simulink model "ec_fixed_slm_hardcode"  (Simulink 10.0)
settings: Solver=FixedStepDiscrete  StartTime=0.0  StopTime=10  RelTol=1e-3
libraries: dspsrcs4 x14, simulink x8, dspsnks4 x4, dspsigops x2, dspbuff3 x2, dspadpt3 x1
settings Model: Creator=Kerry Schutz  LastModifiedBy=bhisma
settings DataIOCC: LimitDataPoints=on  SignalLoggingSaveFormat=ModelDataLogs
settings OptimizationCC: BlockReduction=off  DefaultParameterBehavior=Inlined  InlineInvariantSignals=on  ExpressionDepthLimit=2147483647  StateBitsets=on  DataBitsets=on  ZeroExternalMemoryAtStartup=off  ZeroInternalMemoryAtStartup=off  EfficientFloat2IntCast=on  LifeSpan=1  EfficientTunableParamExpr=on
settings DebuggingCC: AlgebraicLoopMsg=none  SaveWithParameterizedLinksMsg=none  SolverPrmCheckMsg=warning  FcnCallInpInsideContextMsg=warning  StateNameClashWarn=warning
settings HardwareCC: ProdBitPerInt=16  ProdBitPerPointer=16  ProdBitPerSizeT=16  ProdBitPerPtrDiffT=16  ProdIntDivRoundTo=Zero  ProdEndianess=LittleEndian  ProdWordSize=16  ProdHWDeviceType=Microchip->dsPIC  TargetBitPerInt=16  TargetIntDivRoundTo=Zero  TargetEndianess=LittleEndian  TargetWordSize=16  TargetHWDeviceType=Microchip->dsPIC
settings SFSimCC: SimUseLocalCustomCode=on  SimParseCustomCode=off  MATLABDynamicMemAlloc=off  CustomCodeUndefinedFunction=FilterOut
settings RTWCC: Description=Real-Time Workshop Embedded Coder (no auto configuration)  SystemTargetFile=ert.tlc  GenCodeOnly=on  TemplateMakefile=ert_default_tmf  RTWUseLocalCustomCode=on  PortableWordSizes=on  CreateSILPILBlock=SIL
settings CodeAppCC: IgnoreCustomStorageClasses=off  CustomSymbolStrType=$N$R$M  InternalIdentifier=Classic  InlinedPrmAccess=Macros
settings ERTTargetCC: TargetFcnLib=ansi_tfl_tmw.mat  GenerateSampleERTMain=on  IncludeMdlTerminateFcn=off  SupportAbsoluteTime=off  PurelyIntegerCode=on  SupportNonFinite=off  SupportComplex=off  InlinedParameterPlacement=NonHierarchical  ERTCustomFileTemplate=example_file_process.tlc  ConvertIfToSwitch=off  SuppressUnreachableDefaultCases=off

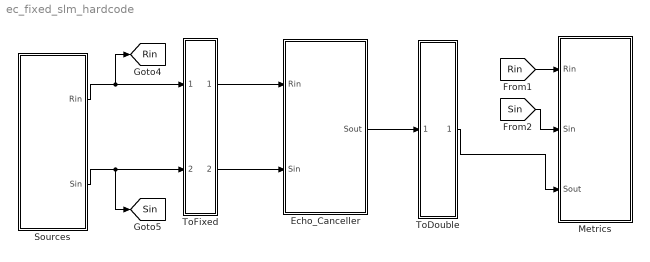
== system ec_fixed_slm_hardcode ==
  Echo_Canceller : Subsystem
  Metrics : Subsystem  TreatAsAtomicUnit=on
  Sources : Subsystem
  ToDouble : Subsystem
  ToFixed : Subsystem
  tag scope: Rin=global, Sin=global
  wires:
  ToFixed/1(Rin) -> Echo_Canceller/1(Rin)
  ToFixed/2(Sin) -> Echo_Canceller/2("Sin ")
  Echo_Canceller/1(Sout) -> ToDouble/1(In2)
  Sources/2(Sin) -> ToFixed/2(" In2"), [Sin]
  Sources/1(Rin) -> ToFixed/1(In1), [Rin]
  [Rin] -> Metrics/1(Rin)
  [Sin] -> Metrics/2(Sin)
  ToDouble/1(Sout) -> Metrics/3(Sout)

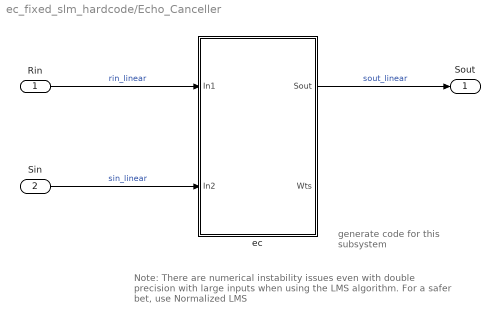
== system ec_fixed_slm_hardcode/Echo_Canceller ==
  note: Note:
      | There are numerical instability issues even with double precision
      | with large inputs when using the LMS algorithm.
      | For a safer bet, use Normalized LMS
  note: generate code for this
      | subsystem
  Rin : Inport
  "Sin " : Inport  Port=2
  ec : Subsystem
  Sout : Outport
  wires:
  Rin/1 -> ec/1(In1)  "rin_linear"
  "Sin "/1 -> ec/2(In2)  "sin_linear"
  ec/1(Sout) -> Sout/1  "sout_linear"

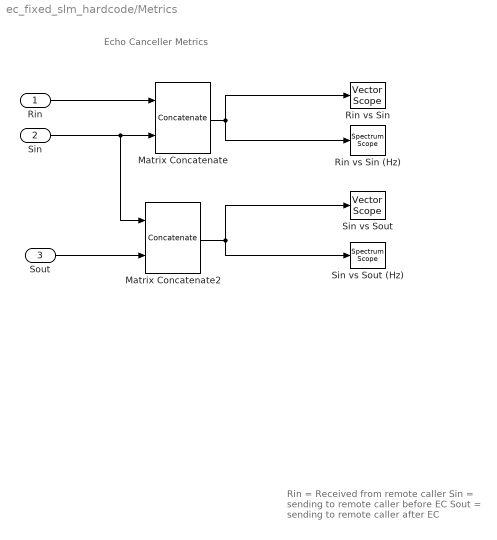
== system ec_fixed_slm_hardcode/Metrics ==
  note: Rin = Received from remote caller
      | Sin = sending to remote caller before EC
      | Sout = sending to remote caller after EC
  note: Echo Canceller Metrics
  Rin : Inport
  Sin : Inport  Port=2
  Sout : Inport  Port=3
  Matrix Concatenate : Concatenate  Mode=Multidimensional array  ConcatenateDimension=2
  Matrix Concatenate2 : Concatenate  Mode=Multidimensional array  ConcatenateDimension=2
  Rin vs Sin : dspsnks4/Vector Scope  ScopeProperties=on  Domain=Time  HorizSpan=1  DisplayProperties=off  AxisGrid=on  Memory=off  FrameNumber=on  AxisLegend=off  AxisZoom=off  OpenScopeAtSimStart=on  OpenScopeImmediately=off  FigPos=[21 752 407 182]  AxisProperties=off  XUnits=Hertz  XRange=[0...Fs/2]  InheritXIncr=on  XIncr=1  XLabel=Time  XLimit=Auto  XMin=0  XMax=1  XStart=0  YUnits=dB  YLabel=Amplitude  LineProperties=off  LineColors=[1 0 0]|[0 1 0]
      settings: SourceProductName=DSP System Toolbox  SourceProductBaseCode=DS  YMin=-1  YMax=1
  Rin vs Sin (Hz) : dspsnks4/Spectrum Scope  SystemSampleTime=-1  ScopeProperties=on  Domain=Frequency  HorizSpan=1  UseBuffer=on  BufferSize=512  Overlap=64  inpFftLenInherit=off  FFTlength=128  numAvg=2  DisplayProperties=off  AxisGrid=on  Memory=off  FrameNumber=on  AxisLegend=off  AxisZoom=off  OpenScopeAtSimStart=on  OpenScopeImmediately=off  FigPos=[22 519 408 178]  AxisProperties=off  XUnits=Hertz  XRange=[0...Fs/2]  InheritXIncr=on  XIncr=1.0  XLabel=Samples  XLimit=Auto  YUnits=dB  XMax=1  XMin=0  YLabel=Magnitude-squared, dB  LineProperties=off  LineColors=[1 0 0]|[0 1 0]  wintypeSpecScope=Hann  RsSpecScope=50  betaSpecScope=5  winsampSpecScope=Periodic
      settings: SourceProductName=DSP System Toolbox  SourceProductBaseCode=DS  YMin=-87.2863320440191  YMax=22.6100164436924
  Sin vs Sout : dspsnks4/Vector Scope  ScopeProperties=on  Domain=Time  HorizSpan=1  DisplayProperties=off  AxisGrid=on  Memory=off  FrameNumber=on  AxisLegend=off  AxisZoom=off  OpenScopeAtSimStart=on  OpenScopeImmediately=off  FigPos=[439 284 406 181]  AxisProperties=off  XUnits=Hertz  XRange=[0...Fs/2]  InheritXIncr=on  XIncr=1  XLabel=Time  XLimit=Auto  XMin=0  XMax=1  XStart=0  YUnits=dB  YLabel=Amplitude  LineProperties=off  LineColors=[1 0 0]|[0 1 0]
      settings: SourceProductName=DSP System Toolbox  SourceProductBaseCode=DS  YMin=-1.10854137455551  YMax=1.10983865900285
  Sin vs Sout (Hz) : dspsnks4/Spectrum Scope  SystemSampleTime=-1  ScopeProperties=on  Domain=Frequency  HorizSpan=1  UseBuffer=on  BufferSize=512  Overlap=64  inpFftLenInherit=off  FFTlength=128  numAvg=2  DisplayProperties=off  AxisGrid=on  Memory=off  FrameNumber=on  AxisLegend=off  AxisZoom=off  OpenScopeAtSimStart=on  OpenScopeImmediately=off  FigPos=[440 519 404 181]  AxisProperties=off  XUnits=Hertz  XRange=[0...Fs/2]  InheritXIncr=on  XIncr=1.0  XLabel=Samples  XLimit=Auto  YUnits=dB  XMax=1  XMin=0  YLabel=Magnitude-squared, dB  LineProperties=off  LineColors=[1 0 0]|[0 1 0]  wintypeSpecScope=Hann  RsSpecScope=50  betaSpecScope=5  winsampSpecScope=Periodic
      settings: SourceProductName=DSP System Toolbox  SourceProductBaseCode=DS  YMin=-128.562839071617  YMax=21.0948472865104
  wires:
  Sout/1 -> Matrix Concatenate2/2
  Matrix Concatenate2/1 -> Sin vs Sout/1, Sin vs Sout (Hz)/1
  Matrix Concatenate/1 -> Rin vs Sin/1, Rin vs Sin (Hz)/1
  Rin/1 -> Matrix Concatenate/1
  Sin/1 -> Matrix Concatenate/2, Matrix Concatenate2/1

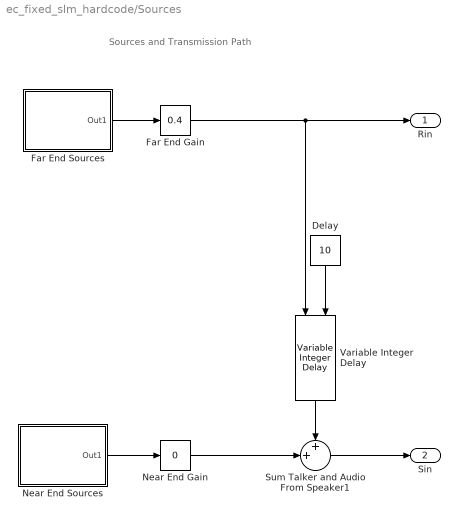
== system ec_fixed_slm_hardcode/Sources ==
  note: Sources and Transmission Path
  Delay : Constant  Value=10  SampleTime=80/8000
  Far End Gain : simulink/Math Operations/Slider Gain  SystemSampleTime=-1  low=0  gain=0.4  high=10
  Far End Sources : Subsystem
  Near End Gain : simulink/Math Operations/Slider Gain  SystemSampleTime=-1  low=0  gain=0  high=10
  Near End Sources : Subsystem
  Sum Talker and Audio From Speaker1 : Sum  Inputs=++|  SaturateOnIntegerOverflow=on  InputSameDT=on  OutDataTypeStr=Inherit: Same as first input
  Variable Integer Delay : dspsigops/Variable Integer Delay  dmax=100  ic=0
      settings: SourceProductName=DSP System Toolbox  SourceProductBaseCode=DS
  Rin : Outport
  Sin : Outport  Port=2
  wires:
  Far End Gain/1 -> Rin/1, Variable Integer Delay/1
  Near End Gain/1 -> Sum Talker and Audio From Speaker1/2
  Near End Sources/1(Out1) -> Near End Gain/1
  Far End Sources/1(Out1) -> Far End Gain/1
  Sum Talker and Audio From Speaker1/1 -> Sin/1
  Variable Integer Delay/1 -> Sum Talker and Audio From Speaker1/1
  Delay/1 -> Variable Integer Delay/2

== system ec_fixed_slm_hardcode/ToDouble ==
  In2 : Inport
  " 6" : DataTypeConversion  OutDataTypeStr=double
  Sout : Outport
  wires:
  In2/1 -> " 6"/1
  " 6"/1 -> Sout/1

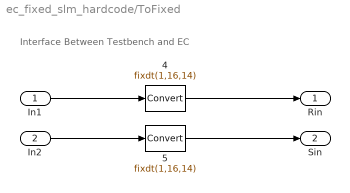
== system ec_fixed_slm_hardcode/ToFixed ==
  note: Interface Between Testbench and EC
  In1 : Inport
  " In2" : Inport  Port=2
  " 4" : DataTypeConversion  OutDataTypeStr=fixdt(1,16,14)
  " 5" : DataTypeConversion  OutDataTypeStr=fixdt(1,16,14)
  Rin : Outport
  Sin : Outport  Port=2
  wires:
  In1/1 -> " 4"/1
  " In2"/1 -> " 5"/1
  " 4"/1 -> Rin/1
  " 5"/1 -> Sin/1

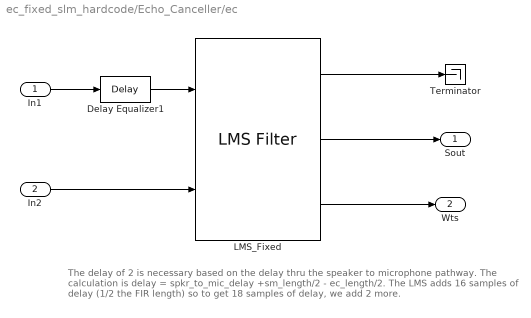
== system ec_fixed_slm_hardcode/Echo_Canceller/ec ==
  note: The delay of 2 is necessary based on the delay thru the speaker to microphone pathway.
      | The calculation is delay = spkr_to_mic_delay +sm_length/2 - ec_length/2. The LMS
      | adds 16 samples of delay (1/2 the FIR length) so to get 18 samples of delay, we add 2 more.
  In1 : Inport
  In2 : Inport  Port=2
  Delay Equalizer1 : dspsigops/Delay  dly_unit=Samples  delay=2  ic_detail=off  dif_ic_for_ch=off  dif_ic_for_dly=off  ic=0  reset_popup=None
      settings: SourceProductName=DSP System Toolbox  SourceProductBaseCode=DS
  LMS_Fixed : dspadpt3/LMS Filter  Algo=LMS  L=32  stepflag=Dialog  mu=300/32768  leakage=1  ic=0  Adapt=off  resetflag=None  weights=on  secondCoeffMode=User-defined  secondCoeffWordLength=2  secondCoeffFracLength=14  accumMode=Binary point scaling  accumWordLength=16  accumFracLength=20  accum2Mode=User-defined  accum2FracLength=15  prodOutputMode=Binary point scaling  prodOutputWordLength=16  prodOutputFracLength=20  prodOutput2Mode=User-defined  prodOutput2FracLength=15  prodOutput3Mode=User-defined  prodOutput3FracLength=15  prodOutput4Mode=User-defined  prodOutput4FracLength=15  quotientMode=User-defined  quotientFracLength=20  memoryMode=Binary point scaling  memoryWordLength=16  memoryFracLength=15  roundingMode=Nearest  overflowMode=off  addnparflag=off
      settings: SourceProductName=DSP System Toolbox  SourceProductBaseCode=DS
  Terminator : Terminator
  Sout : Outport
  Wts : Outport  Port=2
  wires:
  Delay Equalizer1/1 -> LMS_Fixed/1
  LMS_Fixed/3 -> Wts/1
  LMS_Fixed/2 -> Sout/1
  In2/1 -> LMS_Fixed/2
  LMS_Fixed/1 -> Terminator/1
  In1/1 -> Delay Equalizer1/1

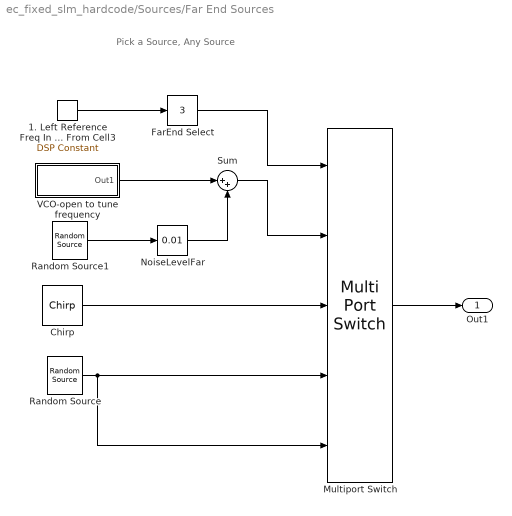
== system ec_fixed_slm_hardcode/Sources/Far End Sources ==
  note: Pick a Source, Any Source
  1. Left Reference Freq In Hz From Cell3 : dspsrcs4/DSP Constant  SystemSampleTime=-1  Value=1  SampleMode=Discrete  discreteOutput=Sample-based  continuousOutput=Sample-based  sampTime=1/8000  framePeriod=2  dataType=double  isSigned=on  wordLen=16  udDataType=sfix(16)  fracBitsMode=Best precision  numFracBits=15  InterpretAs1D=-inf  Ts=-inf  FramebasedOutput=-inf
      settings: SourceProductName=DSP System Toolbox  SourceProductBaseCode=DS  additionalParams=on
  Chirp : dspsrcs4/Chirp  sweep=Linear  mode=Unidirectional  f0=100  f1=4000  t1=80/8000  Tsweep=80/8000  phase=0  Ts=1/8000  spf=80  datatype=Double
      settings: SourceProductName=DSP System Toolbox
  FarEnd Select : simulink/Math Operations/Slider Gain  SystemSampleTime=-1  low=0  gain=3  high=10
  Multiport Switch : MultiPortSwitch  Inputs=4  SampleTime=80/8000
  NoiseLevelFar : simulink/Math Operations/Slider Gain  SystemSampleTime=-1  low=0  gain=0.01  high=1
  Random Source : dspsrcs4/Random Source  SrcType=Gaussian  NormMethod=Ziggurat  CltLength=12  MinVal=0  MaxVal=1  MeanVal=0  VarVal=1  RepMode=Repeatable  rawSeed=1  IsInherit=off  SampMode=Discrete  SampTime=1/8000  SampFrame=80  DataType=Double  OutComplex=Real
  Random Source1 : dspsrcs4/Random Source  SrcType=Gaussian  NormMethod=Ziggurat  CltLength=12  MinVal=0  MaxVal=1  MeanVal=0  VarVal=1  RepMode=Not repeatable  rawSeed=1  IsInherit=off  SampMode=Discrete  SampTime=1/8000  SampFrame=80  DataType=Double  OutComplex=Real
  Sum : Sum  Inputs=|++
  VCO-open to tune frequency : Subsystem
  Out1 : Outport
  wires:
  VCO-open to tune frequency/1(Out1) -> Sum/1
  Multiport Switch/1 -> Out1/1
  Chirp/1 -> Multiport Switch/3
  Random Source/1 -> Multiport Switch/4, Multiport Switch/5
  1. Left Reference Freq In Hz From Cell3/1 -> FarEnd Select/1
  FarEnd Select/1 -> Multiport Switch/1
  Sum/1 -> Multiport Switch/2
  Random Source1/1 -> NoiseLevelFar/1
  NoiseLevelFar/1 -> Sum/2

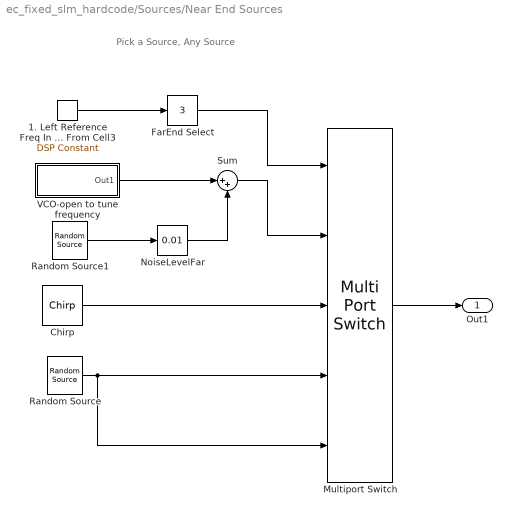
== system ec_fixed_slm_hardcode/Sources/Near End Sources ==
  note: Pick a Source, Any Source
  1. Left Reference Freq In Hz From Cell3 : dspsrcs4/DSP Constant  SystemSampleTime=-1  Value=1  SampleMode=Discrete  discreteOutput=Sample-based  continuousOutput=Sample-based  sampTime=1/8000  framePeriod=2  dataType=double  isSigned=on  wordLen=16  udDataType=sfix(16)  fracBitsMode=Best precision  numFracBits=15  InterpretAs1D=-inf  Ts=-inf  FramebasedOutput=-inf
      settings: SourceProductName=DSP System Toolbox  SourceProductBaseCode=DS  additionalParams=on
  Chirp : dspsrcs4/Chirp  sweep=Linear  mode=Unidirectional  f0=100  f1=4000  t1=80/8000  Tsweep=80/8000  phase=0  Ts=1/8000  spf=80  datatype=Double
      settings: SourceProductName=DSP System Toolbox
  FarEnd Select : simulink/Math Operations/Slider Gain  SystemSampleTime=-1  low=0  gain=3  high=10
  Multiport Switch : MultiPortSwitch  Inputs=4  SampleTime=80/8000
  NoiseLevelFar : simulink/Math Operations/Slider Gain  SystemSampleTime=-1  low=0  gain=0.01  high=1
  Random Source : dspsrcs4/Random Source  SrcType=Gaussian  NormMethod=Ziggurat  CltLength=12  MinVal=0  MaxVal=1  MeanVal=0  VarVal=1  RepMode=Repeatable  rawSeed=1  IsInherit=off  SampMode=Discrete  SampTime=1/8000  SampFrame=80  DataType=Double  OutComplex=Real
  Random Source1 : dspsrcs4/Random Source  SrcType=Gaussian  NormMethod=Ziggurat  CltLength=12  MinVal=0  MaxVal=1  MeanVal=0  VarVal=1  RepMode=Not repeatable  rawSeed=1  IsInherit=off  SampMode=Discrete  SampTime=1/8000  SampFrame=80  DataType=Double  OutComplex=Real
  Sum : Sum  Inputs=|++
  VCO-open to tune frequency : Subsystem
  Out1 : Outport
  wires:
  NoiseLevelFar/1 -> Sum/2
  Random Source1/1 -> NoiseLevelFar/1
  Sum/1 -> Multiport Switch/2
  FarEnd Select/1 -> Multiport Switch/1
  1. Left Reference Freq In Hz From Cell3/1 -> FarEnd Select/1
  Random Source/1 -> Multiport Switch/5, Multiport Switch/4
  Chirp/1 -> Multiport Switch/3
  Multiport Switch/1 -> Out1/1
  VCO-open to tune frequency/1(Out1) -> Sum/1

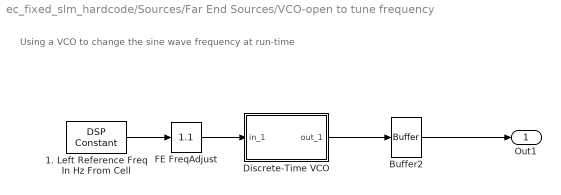
== system ec_fixed_slm_hardcode/Sources/Far End Sources/VCO-open to tune frequency ==
  note: Using a VCO to change the sine wave frequency at run-time
  1. Left Reference Freq In Hz From Cell : dspsrcs4/DSP Constant  SystemSampleTime=-1  Value=1000  SampleMode=Discrete  discreteOutput=Sample-based  continuousOutput=Sample-based  sampTime=1/8000  framePeriod=2  dataType=double  isSigned=on  wordLen=16  udDataType=sfix(16)  fracBitsMode=Best precision  numFracBits=15  InterpretAs1D=-inf  Ts=-inf  FramebasedOutput=-inf
      settings: SourceProductName=DSP System Toolbox  SourceProductBaseCode=DS  additionalParams=on
  Buffer2 : dspbuff3/Buffer  N=80  V=0  ic=0
      settings: SourceProductName=DSP System Toolbox  SourceProductBaseCode=DS
  Discrete-Time VCO : Subsystem  mask(Discrete-Time VCO){Ac=1, Fc=0, Kc=1, Ph=pi/2, ts=1/8000}
      mask prompts: Ac "Output amplitude:"; Fc "Oscillation frequency (Hz):"; Kc "Input sensitivity:"; Ph "Initial phase (rad):"; ts "Sample time:"
      mask help: Generate a discrete-time output signal whose frequency changes in response to the amplitude variations of the input signal. The input signal must be a scalar.
      mask init:
      | if ((length(Ac)~=1) | (length(Fc)~=1) | (length(Kc)~=1) | (length(Ph)~=1) | (length(ts)~=1) |(length(Ph)~=1))error('Mask parameters must be scalar values.');end;
      | pi2=2*pi;
      mask Help: helpview(commbhelp)
      mask Display: disp('Discrete-Time\nVCO (rab)')
  FE FreqAdjust : simulink/Math Operations/Slider Gain  SystemSampleTime=-1  low=0  gain=1.1  high=5
  Out1 : Outport
  wires:
  Buffer2/1 -> Out1/1
  Discrete-Time VCO/1(out_1) -> Buffer2/1
  FE FreqAdjust/1 -> Discrete-Time VCO/1(in_1)
  1. Left Reference Freq In Hz From Cell/1 -> FE FreqAdjust/1

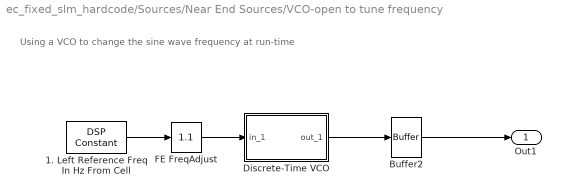
== system ec_fixed_slm_hardcode/Sources/Near End Sources/VCO-open to tune frequency ==
  note: Using a VCO to change the sine wave frequency at run-time
  1. Left Reference Freq In Hz From Cell : dspsrcs4/DSP Constant  SystemSampleTime=-1  Value=1000  SampleMode=Discrete  discreteOutput=Sample-based  continuousOutput=Sample-based  sampTime=1/8000  framePeriod=2  dataType=double  isSigned=on  wordLen=16  udDataType=sfix(16)  fracBitsMode=Best precision  numFracBits=15  InterpretAs1D=-inf  Ts=-inf  FramebasedOutput=-inf
      settings: SourceProductName=DSP System Toolbox  SourceProductBaseCode=DS  additionalParams=on
  Buffer2 : dspbuff3/Buffer  N=80  V=0  ic=0
      settings: SourceProductName=DSP System Toolbox  SourceProductBaseCode=DS
  Discrete-Time VCO : Subsystem  mask(Discrete-Time VCO){Ac=1, Fc=0, Kc=1, Ph=pi/2, ts=1/8000}
      mask prompts: Ac "Output amplitude:"; Fc "Oscillation frequency (Hz):"; Kc "Input sensitivity:"; Ph "Initial phase (rad):"; ts "Sample time:"
      mask help: Generate a discrete-time output signal whose frequency changes in response to the amplitude variations of the input signal. The input signal must be a scalar.
      mask init:
      | if ((length(Ac)~=1) | (length(Fc)~=1) | (length(Kc)~=1) | (length(Ph)~=1) | (length(ts)~=1) |(length(Ph)~=1))error('Mask parameters must be scalar values.');end;
      | pi2=2*pi;
      mask Help: helpview(commbhelp)
      mask Display: disp('Discrete-Time\nVCO (rab)')
  FE FreqAdjust : simulink/Math Operations/Slider Gain  SystemSampleTime=-1  low=0  gain=1.1  high=5
  Out1 : Outport
  wires:
  1. Left Reference Freq In Hz From Cell/1 -> FE FreqAdjust/1
  FE FreqAdjust/1 -> Discrete-Time VCO/1(in_1)
  Discrete-Time VCO/1(out_1) -> Buffer2/1
  Buffer2/1 -> Out1/1

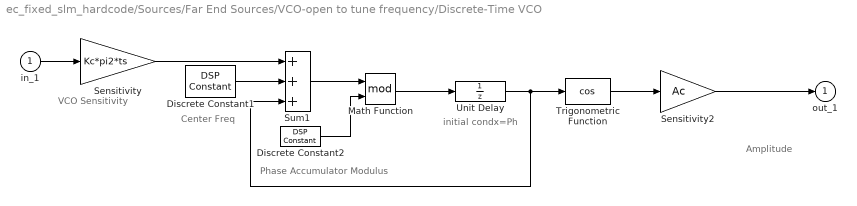
== system ec_fixed_slm_hardcode/Sources/Far End Sources/VCO-open to tune frequency/Discrete-Time VCO ==
  note: Amplitude
  note: Phase Accumulator
      | Modulus
  note: Center Freq
  note: VCO Sensitivity
  note: initial condx=Ph
  in_1 : Inport
  Discrete Constant1 : dspsrcs4/DSP Constant  SystemSampleTime=-1  Value=Fc*pi2*ts  SampleMode=Discrete  discreteOutput=Sample-based (interpret vectors as 1-D)  continuousOutput=Sample-based  sampTime=1/8000  framePeriod=1/8000  dataType=Inherit via back propagation  isSigned=on  wordLen=16  udDataType=sfix(16)  fracBitsMode=Best precision  numFracBits=15  InterpretAs1D=on  Ts=1/8000  FramebasedOutput=off
      settings: SourceProductName=DSP System Toolbox  SourceProductBaseCode=DS  additionalParams=on
  Discrete Constant2 : dspsrcs4/DSP Constant  SystemSampleTime=-1  Value=pi2  SampleMode=Discrete  discreteOutput=Sample-based (interpret vectors as 1-D)  continuousOutput=Sample-based  sampTime=1/8000  framePeriod=1/8000  dataType=Inherit via back propagation  isSigned=on  wordLen=16  udDataType=sfix(16)  fracBitsMode=Best precision  numFracBits=15  InterpretAs1D=on  Ts=1/8000  FramebasedOutput=off
      settings: SourceProductName=DSP System Toolbox  SourceProductBaseCode=DS  additionalParams=on
  Math Function : Math  Operator=mod  SaturateOnIntegerOverflow=on
  Sensitivity : Gain  Gain=Kc*pi2*ts  SaturateOnIntegerOverflow=on  OutDataTypeStr=Inherit: Same as input  ParamDataTypeStr=Inherit: Same as input
  Sensitivity2 : Gain  Gain=Ac  SaturateOnIntegerOverflow=on  OutDataTypeStr=Inherit: Same as input  ParamDataTypeStr=Inherit: Same as input
  Sum1 : Sum  Inputs=+++  SaturateOnIntegerOverflow=on  InputSameDT=on  OutDataTypeStr=Inherit: Same as first input
  Trigonometric Function : Trigonometry  Operator=cos
  Unit Delay : UnitDelay  InitialCondition=Ph  SampleTime=ts
  out_1 : Outport  InitialOutput=0
  wires:
  Discrete Constant1/1 -> Sum1/2
  Sensitivity2/1 -> out_1/1
  Trigonometric Function/1 -> Sensitivity2/1
  Unit Delay/1 -> Trigonometric Function/1, Sum1/3
  Sensitivity/1 -> Sum1/1
  in_1/1 -> Sensitivity/1
  Math Function/1 -> Unit Delay/1
  Sum1/1 -> Math Function/1
  Discrete Constant2/1 -> Math Function/2

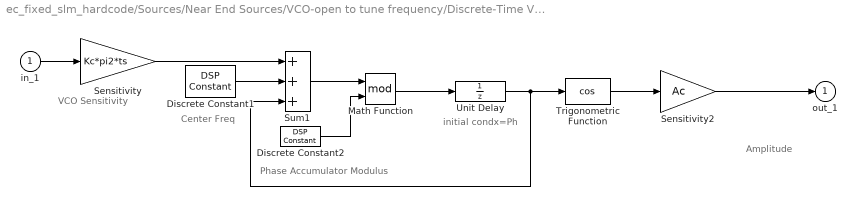
== system ec_fixed_slm_hardcode/Sources/Near End Sources/VCO-open to tune frequency/Discrete-Time VCO ==
  note: initial condx=Ph
  note: VCO Sensitivity
  note: Center Freq
  note: Phase Accumulator
      | Modulus
  note: Amplitude
  in_1 : Inport
  Discrete Constant1 : dspsrcs4/DSP Constant  SystemSampleTime=-1  Value=Fc*pi2*ts  SampleMode=Discrete  discreteOutput=Sample-based (interpret vectors as 1-D)  continuousOutput=Sample-based  sampTime=1/8000  framePeriod=1/8000  dataType=Inherit via back propagation  isSigned=on  wordLen=16  udDataType=sfix(16)  fracBitsMode=Best precision  numFracBits=15  InterpretAs1D=on  Ts=1/8000  FramebasedOutput=off
      settings: SourceProductName=DSP System Toolbox  SourceProductBaseCode=DS  additionalParams=on
  Discrete Constant2 : dspsrcs4/DSP Constant  SystemSampleTime=-1  Value=pi2  SampleMode=Discrete  discreteOutput=Sample-based (interpret vectors as 1-D)  continuousOutput=Sample-based  sampTime=1/8000  framePeriod=1/8000  dataType=Inherit via back propagation  isSigned=on  wordLen=16  udDataType=sfix(16)  fracBitsMode=Best precision  numFracBits=15  InterpretAs1D=on  Ts=1/8000  FramebasedOutput=off
      settings: SourceProductName=DSP System Toolbox  SourceProductBaseCode=DS  additionalParams=on
  Math Function : Math  Operator=mod  SaturateOnIntegerOverflow=on
  Sensitivity : Gain  Gain=Kc*pi2*ts  SaturateOnIntegerOverflow=on  OutDataTypeStr=Inherit: Same as input  ParamDataTypeStr=Inherit: Same as input
  Sensitivity2 : Gain  Gain=Ac  SaturateOnIntegerOverflow=on  OutDataTypeStr=Inherit: Same as input  ParamDataTypeStr=Inherit: Same as input
  Sum1 : Sum  Inputs=+++  SaturateOnIntegerOverflow=on  InputSameDT=on  OutDataTypeStr=Inherit: Same as first input
  Trigonometric Function : Trigonometry  Operator=cos
  Unit Delay : UnitDelay  InitialCondition=Ph  SampleTime=ts
  out_1 : Outport  InitialOutput=0
  wires:
  Discrete Constant2/1 -> Math Function/2
  Sum1/1 -> Math Function/1
  Math Function/1 -> Unit Delay/1
  in_1/1 -> Sensitivity/1
  Sensitivity/1 -> Sum1/1
  Unit Delay/1 -> Sum1/3, Trigonometric Function/1
  Trigonometric Function/1 -> Sensitivity2/1
  Sensitivity2/1 -> out_1/1
  Discrete Constant1/1 -> Sum1/2
